simulink model "WindTurbine_TypeIV_HM"  (R2022a)
settings: Solver=FixedStepDiscrete  StartTime=0  StopTime=3  FixedStep=Ts  RelTol=1e-3  EnableMultiTasking=on
InitFcn:
  | load('xInitial_WPP.mat');
  | Ts = 50e-6;
undefined symbols (not defined in the file): D1, Delta, DiscIntNeverNeededParam, LowerLimit, magnitude, UpperLimit
libraries: powerlib x47, simulink x28, powerlib_meascontrol x17, powerlib_extras x6
(part 1 of 2)
settings Model: SimulationMode=accelerator  Creator=ch0272
settings SolverCC: AlgebraicLoopSolver=TrustRegion
settings DataIOCC: FinalStateName=xInitial_WPP  InitialState=xInitial_WPP  LimitDataPoints=on  LoadInitialState=on  SaveFormat=StructureWithTime  SignalLoggingSaveFormat=ModelDataLogs  ReturnWorkspaceOutputs=off
settings OptimizationCC: ExpressionDepthLimit=2147483647  InitFltsAndDblsToZero=on  LifeSpan=inf
settings DebuggingCC: SaveWithParameterizedLinksMsg=none  UnderspecifiedInitializationDetection=Classic  MergeDetectMultiDrivingBlocksExec=none  SignalResolutionControl=TryResolveAllWithWarning  SolverPrmCheckMsg=warning  MultiTaskCondExecSysMsg=none  FcnCallInpInsideContextMsg=warning  StateNameClashWarn=warning  SFUnexpectedBacktrackingDiag=warning  SFNoUnconditionalDefaultTransitionDiag=warning  ArithmeticOperatorsInVariantConditions=warning
settings HardwareCC: ProdBitPerPointer=32  ProdBitPerSizeT=32  ProdBitPerPtrDiffT=32  ProdLargestAtomicFloat=None  ProdIntDivRoundTo=Undefined  ProdEndianess=Unspecified  ProdWordSize=32  ProdHWDeviceType=32-bit Generic  TargetHWDeviceType=32-bit Generic
settings ModelReferenceCC: PropagateSignalLabelsOutOfModel=off
settings SFSimCC: SimUseLocalCustomCode=off  CustomCodeUndefinedFunction=UseInterfaceOnly
settings RTWCC: Description=General HyperLink Target  SystemTargetFile=hyperlink.tlc  TemplateMakefile=hyperlink.tmf  RTWUseLocalCustomCode=off
settings CodeAppCC: StateflowObjectComments=on
settings STFCustomTargetCC: TargetFcnLib=ansi_tfl_tmw.mat  ModelReferenceCompliant=off  CPPClassGenCompliant=on  SystemTargetFile=hyperlink.tlc
settings GRTTargetCC: TargetFcnLib=ansi_tfl_tmw.mat  TargetLangStandard=C89/C90 (ANSI)  ModelReferenceCompliant=off  ParMdlRefBuildCompliant=off  CompOptLevelCompliant=off  ConcurrentExecutionCompliant=off  CombineOutputUpdateFcns=off  MatFileLogging=off  GRTInterface=on  UseToolchainInfoCompliant=off  ExtModeMexFile=noextcomm
settings ConfigComp: CovMetricSettings=dw  CovSaveCumulativeToWorkspaceVar=on  CovSaveSingleToWorkspaceVar=on  CovExternalEMLEnable=off  CovBoundaryAbsTol=1.0e-5
settings SimscapeCC: SimscapeNormalizeSystem=off

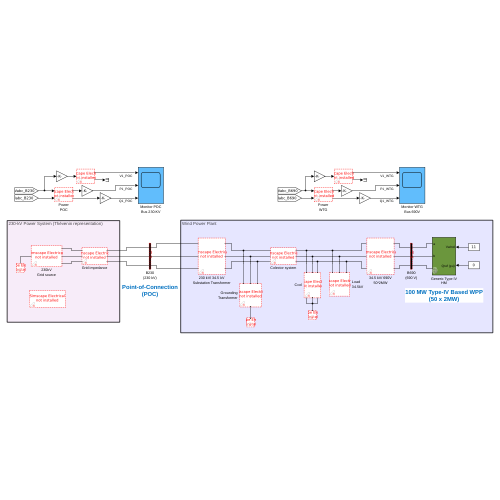
[thumbnail: Simulink's stored preview of the top-level diagram]
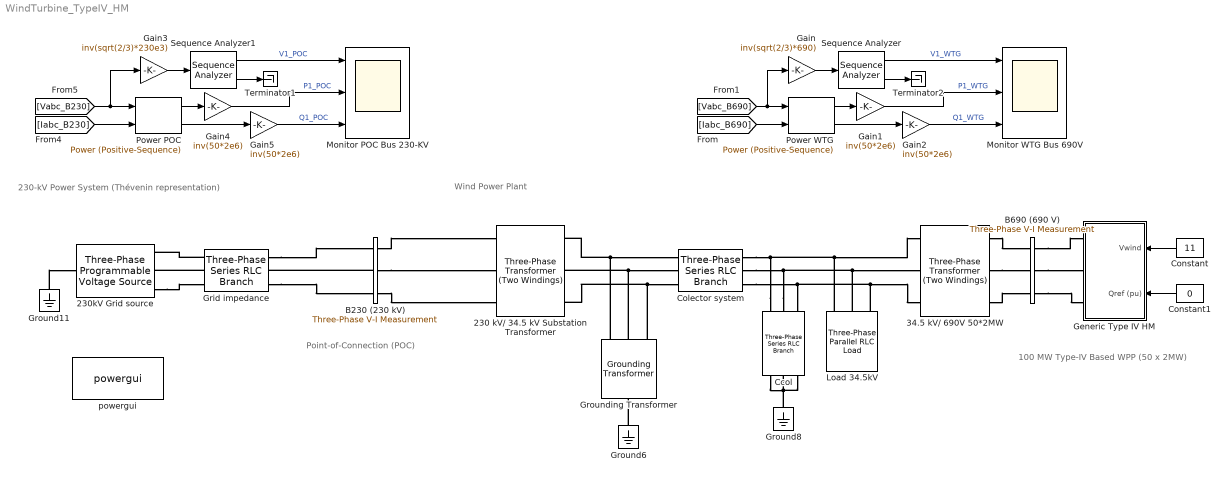
== system WindTurbine_TypeIV_HM ==
  note: 230-kV Power System (Thévenin representation)
  note: Wind Power Plant
  note: 100 MW Type-IV Based WPP
      | (50 x 2MW)
  note: Point-of-Connection
      | (POC)
  230 kV/ 34.5 kV Substation Transformer : powerlib/Elements/Three-Phase Transformer (Two Windings)  Winding1Connection=Yg  Winding2Connection=Delta (D1)  CoreType=Three single-phase transformers  SetSaturation=off  Hysteresis=off  DataFile='hysteresis'  SetInitialFlux=off  Measurements=None  UNITS=pu  NominalPower=[ 115e6 60 ]  Winding1=[230e3 2.25e-3 103.5e-3]  Winding2=[ 34.5e3 0.25e-3 11.5e-3]  Rm=200  Lm=500  L0=0.5  Saturation=[ 0,0 ; 0.002,1 ; 0.01,1.075; 0.025,1.15; 0.05,1.2; 0.1,1.23; 2,1.72 ]  InitialFluxes=[-0.00823815438284101 -0.908209070473327 0.916447224856743]  MoreParameters=off  BreakLoop=off  DataType=off  TransfoNumber=1
  230kV Grid source : powerlib/Electrical Sources/Three-Phase Programmable Voltage Source  PositiveSequence=[230e3 90 60]  VariationEntity=Amplitude  VariationType=Table of time-amplitude pairs  VariationTypeAlt=Step  VariationStep=0.5  VariationRate=10  VariationMagnitude=0.3  VariationFrequency=2  VariationTiming=[1 2]  VariationPhaseA=off  Amplitudes=[1 0.5 1]  TimeValues=[0 1.0 1.1]  HarmonicGeneration=off  HarmonicA=[3 0.2 -25 0]  HarmonicB=[2 0.15 35 2]  Timing="[0.05  3]"  BusType=swing  Pref=0  Qref=0  Qmin=-inf  Qmax=inf
  34.5 kV/ 690V 50*2MW : powerlib/Elements/Three-Phase Transformer (Two Windings)  Winding1Connection=Delta (D1)  Winding2Connection=Yg  CoreType=Three single-phase transformers  SetSaturation=off  Hysteresis=off  DataFile='hysteresis'  SetInitialFlux=off  Measurements=Winding currents  UNITS=pu  NominalPower=[ 115e6 , 60 ]  Winding1=[ 34.5e3 , 3.375e-3 , 51.3e-3]  Winding2=[ 690 , 0.375e-3, 5.7e-3]  Rm=200  Lm=500  L0=0.5  Saturation=[ 0,0 ; 0.002,1 ; 0.01,1.075; 0.025,1.15; 0.05,1.2; 0.1,1.23; 2,1.72 ]  InitialFluxes=[-0.0108935053581042 -0.89679491323339 0.907688418591632]  MoreParameters=off  BreakLoop=off  DataType=off  TransfoNumber=1
  B230 (230 kV) : powerlib/Measurements/Three-Phase V-I Measurement  VoltageMeasurement=phase-to-ground  SetLabelV=on  LabelV=Vabc_B230  Vpu=off  VpuLL=off  CurrentMeasurement=yes  SetLabelI=on  LabelI=Iabc_B230  Ipu=off  Pbase=100e6  Vbase=230e3  OutputType=Complex  PhasorSimulation=off  PSBequivalent=0
  B690 (690 V) : powerlib/Measurements/Three-Phase V-I Measurement  VoltageMeasurement=phase-to-ground  SetLabelV=on  LabelV=Vabc_B690  Vpu=off  VpuLL=off  CurrentMeasurement=yes  SetLabelI=on  LabelI=Iabc_B690  Ipu=off  Pbase=100e6  Vbase=690  OutputType=Complex  PhasorSimulation=off  PSBequivalent=0
  Ccol : powerlib/Elements/Three-Phase Series RLC Branch  LConnTagsString=A|B|C  RConnTagsString=A|B|C  BranchType=C  Resistance=1  Inductance=1e-3  Capacitance=7.17e-6  Measurements=Branch voltages
  Colector system : powerlib/Elements/Three-Phase Series RLC Branch  LConnTagsString=A|B|C  RConnTagsString=A|B|C  BranchType=RL  Resistance=0.22  Inductance=0.391e-3  Capacitance=1e-6  Measurements=Branch currents
  Constant : Constant  Value=11
  Constant1 : Constant  Value=0
  Gain : Gain  Gain=inv(sqrt(2/3)*690)
  Gain{1..2,4..5} (4 alike) : Gain  Gain=inv(50*2e6)
  Gain3 : Gain  Gain=inv(sqrt(2/3)*230e3)
  Generic Type IV HM : Subsystem  mask(WEC Type IV Hybrid Model (HM)){U_rated=690, f_rated=60, FRT_Mode=FRT Mode 1 (I_reactive support), FRT1_triggers=[0.8 1.2 0.01 5], FRT1_k_vrt=[2 2], FRT2_triggers=[0.8 1.2 0.01 5], FRT2_ramp=[0.5 0.2 0], u_protect=[1.25 0.1 0.8 5], f_protect=[1.05 1 0.95 1], Nb_WT=50}
      mask prompts: U_rated "Grid nominal voltage (V):"; f_rated "Grid nominal frequency (Hz):"; FRT_Mode "Fault-ride-through (FRT) Strategy:"; FRT1_triggers "UVRT-trigger, OVRT-trigger, FRT-band (pu) and FRT-maxTime (s):"; FRT1_k_vrt "Proportional gains [k_UVRT k_OVRT]:"; FRT2_triggers "UVRT-trigger, OVRT-trigger, FRT-band (pu) and FRT-maxTime (s):"; FRT2_ramp "P and Q ramp-up times in (s) and start-delay (s):"; u_protect "Voltage protection [Vmax(pu) Vmax_delay(s) Vmin(pu) Vmin_delay(s)]:"; f_protect "Frequency protection [fmax(pu) fmax_delax(s) fmin(pu) fmin_delay(s)]:"; Nb_WT "Number of wind turbines:"
      mask init:
      | %% FRT:
      | if FRT_Mode == 1
      |     u_uvrt = FRT1_triggers(1);
      |     u_ovrt = FRT1_triggers(2);
      |     frt_band = FRT1_triggers(3);
      |     FRT_maxTime = FRT1_triggers(4);
      |     k_uvrt = max(FRT1_k_vrt(1),0); % limit low to 0
      |     k_uvrt = min(FRT1_k_vrt(1),10); % limit max to 10
      |     k_ovrt = max(FRT1_k_vrt(2),0); % limit low to 0
      |     k_ovrt = min(FRT1_k_vrt(2),10); % limit low to 10
      |     FRT2_ramp_p = 0;
      |     FRT2_ramp_q = 0;
      |     FRT2_delay  = 0;
      | elseif FRT_Mode == 2
      |     u_uvrt = FRT2_triggers(1);
      |     u_ovrt = FRT2_triggers(2);
      |     frt_band = FRT2_triggers(3);
      |     FRT_maxTime = FRT2_triggers(4);
      |     FRT2_ramp_p = FRT2_ramp(1);
      |     FRT2_ramp_q = FRT2_ramp(2);
      |     FRT2_delay  = min(FRT2_ramp(3),1); % limt low to 1s
      |     k_uvrt = 0;
      |     k_ovrt = 0;
      | end
      | 
      | %% Protection settings:
      | umax_protection = u_protect(1);
      | umax_delay = u_protect(2);
      | umin_protection = u_protect(3);
      | umin_delay = u_protect(4);
      | fmax_protection = f_protect(1);
      | fmax_delay = f_protect(2);
      | fmin_protection = f_protect(3);
      | fmin_delay = f_protect(4);
      | 
      | %% WEC Parameters:
      | P_rated = 2e6;
      | Q_rated = 1.5e6;
      | i_rated = sqrt(2)*abs((P_rated-j*(Q_rated))/(sqrt(3)*U_rated));
      | i_max = 1.075*i_rated;
      | f_boost = 2e3;
      | f_chopper = 2e3;
      | Vdc_ref = 1250;
      | 
      | %% Generator:
      | % Nominal power, voltage, frequency, field current  [ Pn(VA) Vn(Vrms) fn(Hz) ifn(A) ]:
      | Pgen_nom = 2e6; % [W] 
      | Vgen_nom = 0.83e3; % [V]
      | fgen_nom = 10.8; % [Hz]
      | ifngen_nom = 31.7; % [A]
      | % Stator  [ Rs(ohm)  Ll,Lmd,Lmq(H) ]:
      | Rs_gen = 25e-3; % [Ohm]
      | Ll_gen = 7e-3; % [H]
      | Lmd_gen = 10e-3; % [H]
      | Lmq_gen = 10e-3; % [H]
      | % Field  [ Rf'(ohm)  Llfd'(H) ]:
      | Rf_prime = 3.5e-3; % [Ohm]
      | Llfd_prime = 85e-6; % [H]
      | % Dampers   [ Rkd',Llkd'  Rkq1',Llkq1'  ] (R=ohm,L=H):
      | Rkd_prime = 1e6; % [Ohm]
      | Llkd_prime = 1e-6; % [H]
      | Rkq_prime = 1e6; % [Ohm]
      | Llkq_prime = 1e-6; % [H]
      | % Inertia, friction factor, pole pairs [ J(kg.m^2)  F(N.m.s)  p() ]:
      | J_gen = 7.5e6; % [kgm^2]
      | F_gen = 0; % [Nms]
      | p_gen = 36; % [pole pairs]
      | % Initial conditions  [ dw(%)  th(deg)  ia,ib,ic(A)  pha,phb,phc(deg)  Vf(V) ]:
      | dw_gen = 0; % [%]
      | th_gen = -17.7582; % [deg]
      | ia_gen = 1967.46; % [A]
      | ib_gen = 1967.46; % [A]
      | ic_gen = 1967.46; % [A]
      | pha_gen = 0; % [deg]
      | phb_gen = -120; % [deg]
      | phc_gen = 120; % [deg]
      | Vf_gen = 580; % [V]
      | if0 = 110; % [A]
      | % Load-flow-TAB:
      | Qmax_gen = inf;
      | 
      | %% Universal Bridge (rectifier):
      | Rs_rec = 1e5; % [Ohm]
      | Cs_rec = 1e9; % [F]
      | Ron_rec = 1e-4; % [Ohm]
      | Lon_rec = 0; % [H]
      | Vf_rec = 0; % [V]
      | 
      | %% DC-Link:
      | R1_dc = 1e3; % [Ohm]
      | C1_dc = 50e-3; % [F]
      | C1_V0 = 3*sqrt(2)/pi*830; % [V]
      | R_boost = 10e-3; % [Ohm] 
      | L_boost = 100e-6; % [H]
      | i0_boost = 0; % [A]
      | Ron_igbt_boost = 1e-4; % [Ohm]
      | Lon_igbt_boost = 0; % [H]
      | Vf_igbt_boost = 0; % [V]
      | Rs_igbt_boost = 1e5; % [Ohm]
      | i0_igbt_boost = 0; % [A]
      | Cs_igbt_boost = 1e9; % [F]
      | Ron_diode_boost = 1e-4; % [Ohm]
      | Lon_diode_boost = 0; % [H]
      | Vf_diode_boost = 0; % [V]
      | Rs_diode_boost = 1e5; % [Ohm]
      | Cs_diode_boost = 1e9; % [F]
      | Ron_igbt_chop = 1e-4; % [Ohm]
      | Lon_igbt_chop = 0; % [H]
      | Vf_igbt_chop = 0; % [V]
      | Rs_igbt_chop = 1e5; % [Ohm]
      | Cs_igbt_chop = 1e9; % [F]
      | R_chopper = 0.15; % [Ohm]
      | R2_dc = 1e3; % [Ohm]
      | C2_dc = 0.3; % [F]
      | C2_V0 = 0.9*(Vdc_ref); % [V]
      | Chop_band = 0.025; % [%]
      | 
      | %% Grid Side Converter:
      | Rs_inv = 1e5; % [Ohm]
      | Cs_inv = 1e9; % [F]
      | Ron_inv = 1e-4; % [Ohm]
      | Vf_inv = 0; % [V]
      | Vfd_inv = 0; % [V]
      | 
      | %% Output Filter:
      | L1_filter = 150e-6; % [H]
      | Rshunt_filter = 0.25; % [Ohm]
      | Lshunt_filter = 15e-3; % [H]
      | Cshunt_filter = 1300e-6; % [F]
      | L2_filter = 5e-6; % [H]
      | 
      | %% Three-phase breaker;
      | Ron_breaker = 1e-9; % [Ohm]
      | Rs_breaker = 1e6; % [Ohm]
      | Cs_breaker = 1e9; % [F]
      | 
      | %% Turbine Control:
      | % Rate Limiter (wind speed):
      | v_rise_rate = 5; % m/s
      | v_fall_rate = -5; % m/s
      | v_init = 11;
      | % Pitch_angle:
      | Beta0 = 0; % [deg]
      | % Vdc control:
      | Vdc1_lowLim = 0; % [V]
      | Vdc1_Kp = 0.75; 
      | Vdc1_Ki = 0.075;
      | Vdc1_stateInit = 0.4; 
      | % Wind turbine:
      | R_turb = 42; % [m]
      | ro_air = 1.225; % air density
      | vspeed_max = 11; % [m/s]
      | vspeed_min = 4; % [m/s]
      | lambda_opt = 7.1;
      | w_init = 1.878; % [rad/s]
      | wr_ref_tau = 8; % [s]
      | 
      | %% Extract References:
      | % Measurement Filter (Voltage):
      | f_cut_volt = 10e3; % [Hz]
      | zeta_filt_volt = 1/sqrt(2); % [-]
      | % Measurement Filter (Voltage):
      | f_cut_curr = 10e3; % [Hz]
      | zeta_filt_curr = 1/sqrt(2); % [-]
      | % PLL:
      | pll_Ki = 2.13; % [-]
      | pll_Kp = 0.1775; % [-]
      | 
      | %% Grid-Side Inverter Control:
      | % Vdc2 control:
      | Vdc2_tau = 2*inv(f_rated); % [s]
      | Vdc2_filt_init = C2_V0; % [V]
      | Vdc2_Kp = 10; 
      | Vdc2_Ki = 75; 
      | Vdc2_stateInit = 2000; % [V]
      | % Reactive power control:
      | Q_Kp = 1e-3; % proportional gain
      | Q_Ki = 0.035; % integral gain
      | Q_stateInit = 0; % [V]
      mask Help:
      | Please, refer to work published in:
      | A. S. Trevisan, A. A. El-Deib, R. Gagnon, J. Mahseredjian, and M. Fecteau, “Field Validated Generic EMT-Type Model of a Full Converter Wind Turbine Based on a Gearless Externally Excited Synchronous Generator,” IEEE Trans. Power Deliv., vol. 33, no. 5, pp. 2284–2293, Oct. 2018.
      | 
      | Author: Aramis Schwanka Trevisan
      | aramis.schwanka.trevisan@enercon.de
      mask TypeOptions FRT_Mode: FRT Mode 1 (I_reactive support) | FRT Mode 2 (Zero power mode)
      mask Callback FRT_Mode:
      | BlockName=getfullname(gcb);
      | 
      | Param_Show=get_param(BlockName,'FRT_Mode');
      | Param_Visible=get_param(BlockName,'MaskVisibilities');
      | Param_Visible{3}='on';
      | Param_Visible{4}='off';Param_Visible{5}='off';Param_Visible{6}='off';Param_Visible{7}='off';
      | 
      | switch Param_Show
      | 	case 'FRT Mode 1 (I_reactive support)'
      | 		Param_Visible{4}='on';Param_Visible{5}='on';
      |     case 'FRT Mode 2 (Zero power mode)'
      | 		Param_Visible{6}='on';Param_Visible{7}='on';
      | end
      | 
      | set_param(BlockName,'MaskVisibilities',Param_Visible);
  Grid impedance : powerlib/Elements/Three-Phase Series RLC Branch  LConnTagsString=A|B|C  RConnTagsString=A|B|C  BranchType=RL  Resistance=(230e3^2/800e6)/12.5  Inductance=(230e3^2/800e6)/2/pi/60  Capacitance=1e-6  Measurements=Branch currents
  Ground11 : powerlib/Elements/Ground  LConnTagsString=a
  Ground6 : powerlib/Elements/Ground  LConnTagsString=a
  Ground8 : powerlib/Elements/Ground  LConnTagsString=a
  Grounding Transformer : powerlib/Elements/Grounding Transformer   UNITS=pu  NominalPower="[100e6   60]"  NominalVoltage=34.5e3  ZeroSequenceImpedance_pu=[23.5245 , 630.1197]*1e-3  MagnetizationBranch_pu=[1e6 inf]  ZeroSequenceImpedance_SI=[0.28 7.5]  MagnetizationBranch_SI=[59513 59513]  Measurements=None
  Load 34.5kV : powerlib/Elements/Three-Phase Parallel RLC Load  LConnTagsString=A|B|C  Configuration=Y (grounded)  NominalVoltage=34.5e3  Vabc=[1e3 1e3 1e3]  Vabcp=[1e3 1e3 1e3]  NominalFrequency=60  UnbalancedPower=off  ActivePower=60e3  InductivePower=0  CapacitivePower=0  Pabc=[10e3 9e3 11e3]  QLabc=[100 90 110]  QCabc=[100 90 110]  Pabcp=[10e3 9e3 11e3]  QLabcp=[100 90 110]  QCabcp=[100 90 110]  Measurements=Branch currents  LoadType=constant Z
  Monitor POC Bus 230-KV : Scope  NumInputPorts=3
  Monitor WTG Bus 690V : Scope  NumInputPorts=3
  Power POC : powerlib_meascontrol/Measurements/Power (Positive-Sequence)  Freq=60  Vinit=[0, 0]  Iinit=[0, 0]  Ts=Ts
  Power WTG : powerlib_meascontrol/Measurements/Power (Positive-Sequence)  Freq=60  Vinit=[0, 0]  Iinit=[0, 0]  Ts=Ts
  Sequence Analyzer : powerlib_meascontrol/Measurements/Sequence Analyzer  Freq=60  n=1  seq=Positive  InInit=[1, 0]  Ts=Ts
  Sequence Analyzer1 : powerlib_meascontrol/Measurements/Sequence Analyzer  Freq=60  n=1  seq=Positive  InInit=[1, 0]  Ts=Ts
  Terminator1 : Terminator
  Terminator2 : Terminator
  powergui : powerlib/powergui  SimulationMode=Discrete  SolverType=Tustin  SampleTime=Ts  frequency=60  SPID=off  DisableSnubberDevices=off  DisableRonSwitches=off  DisableVfSwitches=off  SwTol=0  DisplayEquations=off  Interpol=off  ExternalGateDelay=off  methode=off  Ts=0  FunctionMessages=off  echomessages=off  HookPort=off  EnableUseOfTLC=off  x0status=blocks  frequencyindice=0  Pbase=100e6  ErrMax=1e-4  Iterations=50  UnitsV=kV  UnitsW=MW  buscounter=0  RestoreLinks=warning  ResistiveCurrentMeasurement=off  Frange=[1:1:300]  Ylog=off  Xlog=off  ShowGrid=off  save=on  variable=ZData  structure=Vabc_Iabc  ZoomFFT=on  StartTime=0.0  cycles=1  DisplayStyle=1  fundamental=60  FreqAxis=off  MaxFrequency=1000  frequencyindicesteady=1  RmsSteady=1  display=off
  wires:
  Constant1/1 -> Generic Type IV HM/2(Qref (pu))
  Constant/1 -> Generic Type IV HM/1(Vwind)
  [Iabc_B690] -> Power WTG/2
  Power WTG/1 -> Gain1/1
  Power WTG/2 -> Gain2/1
  Sequence Analyzer/2 -> Terminator2/1
  Sequence Analyzer/1 -> Monitor WTG Bus 690V/1  "V1_WTG"
  [Vabc_B690] -> Gain/1, Power WTG/1
  Power POC/1 -> Gain4/1
  Power POC/2 -> Gain5/1
  Sequence Analyzer1/2 -> Terminator1/1
  Sequence Analyzer1/1 -> Monitor POC Bus 230-KV/1  "V1_POC"
  [Vabc_B230] -> Gain3/1, Power POC/1
  [Iabc_B230] -> Power POC/2
  Gain/1 -> Sequence Analyzer/1
  Gain1/1 -> Monitor WTG Bus 690V/2  "P1_WTG"
  Gain2/1 -> Monitor WTG Bus 690V/3  "Q1_WTG"
  Gain3/1 -> Sequence Analyzer1/1
  Gain4/1 -> Monitor POC Bus 230-KV/2  "P1_POC"
  Gain5/1 -> Monitor POC Bus 230-KV/3  "Q1_POC"
  connections:
  Grounding Transformer/LConn1 -- Colector system/RConn1 -- 230 kV/ 34.5 kV Substation Transformer/RConn1
  Ccol/RConn3 -- Ccol/RConn2 -- Ground8/LConn1 -- Ccol/RConn1
  Grounding Transformer/LConn2 -- Colector system/RConn2 -- 230 kV/ 34.5 kV Substation Transformer/RConn2
  Grounding Transformer/LConn3 -- Colector system/RConn3 -- 230 kV/ 34.5 kV Substation Transformer/RConn3
  Load 34.5kV/LConn3 -- Colector system/LConn3 -- Ccol/LConn3 -- 34.5 kV/ 690V 50*2MW/LConn3
  Ccol/LConn2 -- Load 34.5kV/LConn2 -- 34.5 kV/ 690V 50*2MW/LConn2 -- Colector system/LConn2
  Ccol/LConn1 -- Load 34.5kV/LConn1 -- 34.5 kV/ 690V 50*2MW/LConn1 -- Colector system/LConn1
  Ground11/LConn1 -- 230kV Grid source/LConn1
  B690 (690 V)/LConn2 -- Generic Type IV HM/RConn2
  B690 (690 V)/LConn1 -- Generic Type IV HM/RConn1
  B690 (690 V)/LConn3 -- Generic Type IV HM/RConn3
  Ground6/LConn1 -- Grounding Transformer/RConn1
  B230 (230 kV)/LConn2 -- 230 kV/ 34.5 kV Substation Transformer/LConn2
  B230 (230 kV)/LConn1 -- 230 kV/ 34.5 kV Substation Transformer/LConn1
  B230 (230 kV)/LConn3 -- 230 kV/ 34.5 kV Substation Transformer/LConn3
  34.5 kV/ 690V 50*2MW/RConn2 -- B690 (690 V)/RConn2
  34.5 kV/ 690V 50*2MW/RConn1 -- B690 (690 V)/RConn1
  34.5 kV/ 690V 50*2MW/RConn3 -- B690 (690 V)/RConn3
  Grid impedance/RConn2 -- 230kV Grid source/RConn2
  Grid impedance/RConn1 -- 230kV Grid source/RConn1
  230kV Grid source/RConn3 -- Grid impedance/RConn3
  Grid impedance/LConn1 -- B230 (230 kV)/RConn1
  B230 (230 kV)/RConn2 -- Grid impedance/LConn2
  Grid impedance/LConn3 -- B230 (230 kV)/RConn3

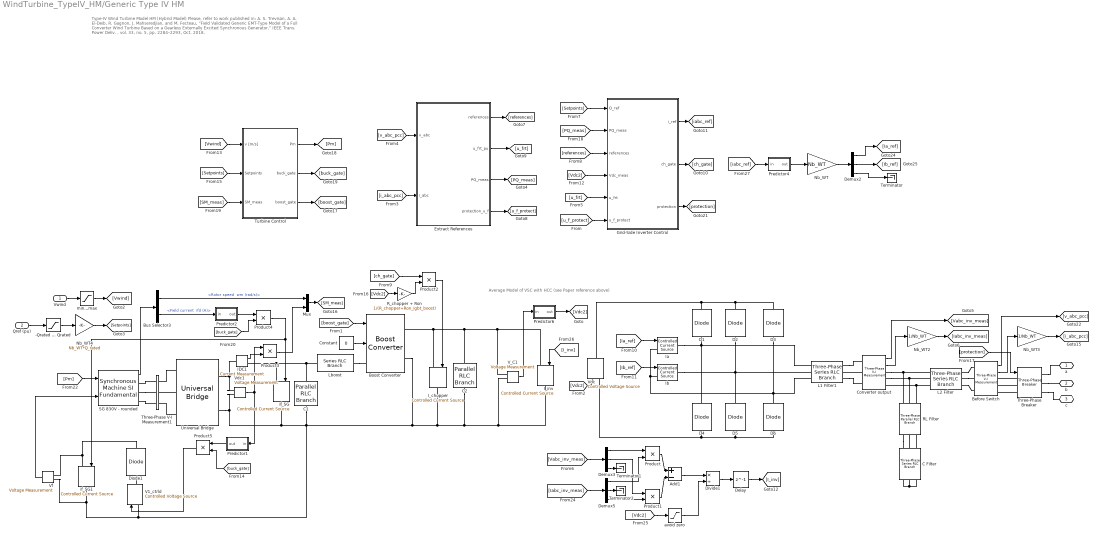
== system WindTurbine_TypeIV_HM/Generic Type IV HM ==
  note: Average Model of VSC with HCC (see Paper reference above)
  note: Type-IV Wind Turbine Model
      | HM (Hybrid Model)
      |
      | Please, refer to work published in:
      |
      | A. S. Trevisan, A. A. El-Deib, R. Gagnon, J. Mahseredjian, and M. Fecteau, “Field Validated Generic EMT-Type Model of a Full Converter Wind Turbine Based on a Gearless Externally Excited Synchronous Generator,” IEEE Trans. Power Deliv. , vol. 33, no. 5, pp. 2284–2293, Oct. 2018.
  Vwind : Inport
  Qref (pu) : Inport  Port=2
  -Qrated ... Qrated : Saturate  UpperLimit=1  LowerLimit=-1
  Add1 : Sum  Inputs=+-
  Before Switch : powerlib/Measurements/Three-Phase V-I Measurement  VoltageMeasurement=phase-to-ground  SetLabelV=off  LabelV=Vabc  Vpu=off  VpuLL=off  CurrentMeasurement=yes  SetLabelI=off  LabelI=Iabc  Ipu=off  Pbase=100e6  Vbase=500e3  OutputType=Complex  PhasorSimulation=off  PSBequivalent=0
  Boost Converter : powerlib/Power Electronics/Boost Converter  ModelType=Switching function  Ron=1e-3  Rs=1e6  Cs=inf  Vforward=[0,0]  Ron_Diode=Ron_diode_boost  Rs_Diode=Rs_diode_boost  Cs_Diode=Cs_diode_boost  Vf_Diode=Vf_diode_boost  Rs_CurrentSource=1e5
  Bus Selector3 : BusSelector  OutputSignals="Mechanical.Rotor speed  wm (rad/s),dq0 components.Field current  ifd (A)"
  C Filter : powerlib/Elements/Three-Phase Series RLC Branch  LConnTagsString=A|B|C  RConnTagsString=A|B|C  BranchType=C  Resistance=1  Inductance=50e-6  Capacitance=Cshunt_filter*Nb_WT  Measurements=Branch voltages
  C1 : powerlib/Elements/Parallel RLC Branch  LConnTagsString=a  RConnTagsString=__new0  BranchType=C  Resistance=R1_dc  Inductance=1e-3  SetiL0=off  InitialCurrent=0  Capacitance=C1_dc  Setx0=on  InitialVoltage=C1_V0  Measurements=None
  C2 : powerlib/Elements/Parallel RLC Branch  LConnTagsString=a  RConnTagsString=__new0  BranchType=C  Resistance=R2_dc  Inductance=1e-3  SetiL0=off  InitialCurrent=0  Capacitance=C2_dc  Setx0=on  InitialVoltage=C2_V0  Measurements=None
  Constant : Constant  Value=0
  Converter output : powerlib/Measurements/Three-Phase V-I Measurement  VoltageMeasurement=phase-to-phase  SetLabelV=off  LabelV=Vabc  Vpu=off  VpuLL=off  CurrentMeasurement=yes  SetLabelI=off  LabelI=Iabc  Ipu=off  Pbase=100e6  Vbase=500e3  OutputType=Complex  PhasorSimulation=off  PSBequivalent=0
  D{1..6} (6 alike) : powerlib/Power Electronics/Diode  Ron=Ron_inv/Nb_WT  Lon=0  Vf=Vfd_inv  IC=0  UseSnubber=off  Rs=Rs_inv/Nb_WT  Cs=Cs_inv*Nb_WT  Measurements=off
  Delay : Delay  DelayLength=1  SampleTime=Ts
  Demux2 : Demux  Outputs=3
  Demux3 : Demux  Outputs=3
  Demux5 : Demux  Outputs=3
  Diode1 : powerlib/Power Electronics/Diode  Ron=1e-3  Lon=0  Vf=0  IC=0  UseSnubber=off  Rs=1e5  Cs=250e-9  Measurements=off
  Divide1 : Product  Inputs=*/
  Extract References : Subsystem
  Grid-Side Inverter Control : Subsystem
  IDC1 : powerlib/Measurements/Current Measurement  PhasorSimulation=off  OutputType=Complex  PSBequivalent=0
  I_chopper : powerlib/Electrical Sources/Controlled Current Source  Initialize=on  Source_Type=AC  Amplitude=0  Phase=0  Frequency=0  Measurements=None
  I_inv : powerlib/Electrical Sources/Controlled Current Source  Initialize=on  Source_Type=AC  Amplitude=0  Phase=0  Frequency=0  Measurements=None
  Ia : powerlib/Electrical Sources/Controlled Current Source  Initialize=on  Source_Type=AC  Amplitude=0  Phase=0  Frequency=0  Measurements=None
  Ib : powerlib/Electrical Sources/Controlled Current Source  Initialize=on  Source_Type=AC  Amplitude=0  Phase=0  Frequency=0  Measurements=None
  L1 Filter1 : powerlib/Elements/Three-Phase Series RLC Branch  LConnTagsString=A|B|C  RConnTagsString=A|B|C  BranchType=L  Resistance=1  Inductance=L1_filter/Nb_WT  Capacitance=1e-6  Measurements=None
  L2 Filter : powerlib/Elements/Three-Phase Series RLC Branch  LConnTagsString=A|B|C  RConnTagsString=A|B|C  BranchType=L  Resistance=1  Inductance=L2_filter/Nb_WT  Capacitance=1e-6  Measurements=None
  Lboost : powerlib/Elements/Series RLC Branch  LConnTagsString=__new0  RConnTagsString=__new0  BranchType=RL  Resistance=R_boost  Inductance=L_boost  SetiL0=on  InitialCurrent=i0_boost  Capacitance=100e-6  Setx0=on  InitialVoltage=350  Measurements=None
  Mux : Mux  Inputs=2
  Nb_WT : Gain  Gain=Nb_WT
  Nb_WT2 : Gain  Gain=1/Nb_WT
  Nb_WT3 : Gain  Gain=1/Nb_WT
  Nb_WT4 : Gain  Gain=Nb_WT*Q_rated
  Predictor1 : Subsystem  mask{Init_value=3*sqrt(2)/pi*830, Ts=Ts}
      mask prompts: Init_value "Initial value:"; Ts "Sample time (Ts):"
  Predictor2 : Subsystem  mask{Init_value=if0, Ts=Ts}
      mask prompts: Init_value "Initial value:"; Ts "Sample time (Ts):"
  Predictor4 : Subsystem  mask{Init_value=0, Ts=Ts}
      mask prompts: Init_value "Initial value:"; Ts "Sample time (Ts):"
  Predictor6 : Subsystem  mask{Init_value=0.9*(Vdc_ref), Ts=Ts}
      mask prompts: Init_value "Initial value:"; Ts "Sample time (Ts):"
  Product{,1..5} (6 alike) : Product
  RL Filter : powerlib/Elements/Three-Phase Parallel RLC Branch  LConnTagsString=A|B|C  RConnTagsString=A|B|C  BranchType=RL  Resistance=Rshunt_filter/Nb_WT  Inductance=Lshunt_filter/Nb_WT  Capacitance=1e-6  Measurements=Branch currents
  R_chopper + Ron : Gain  Gain=1/(R_chopper+Ron_igbt_boost)
  SG 830V - rounded : powerlib/Machines/Synchronous Machine SI Fundamental  PresetModel=No  MechanicalLoad=Mechanical power Pm  ShowDetailedParameters=on  RotorType=Salient-pole  Units=SI fundamental parameters  MeasurementBus=off  NominalParameters="[ Pgen_nom  Vgen_nom  fgen_nom  ifngen_nom]"  Stator=[ Rs_gen Ll_gen Lmd_gen Lmq_gen ]  Field=[ Rf_prime Llfd_prime ]  Dampers2=[ 0.0664, 1.387e-3, 0.0292, 6.896e-4, 7.907e-3, 2.477e-3]  Dampers1=[ Rkd_prime Llkd_prime Rkq_prime Llkq_prime ]  Mechanical=[ J_gen F_gen p_gen ]  PolePairs=36  InitialConditions=[ dw_gen th_gen ia_gen ib_gen ic_gen pha_gen phb_gen phc_gen Vf_gen ]  SetSaturation=off  Saturation=[695.64,774.7,917.5,1001.6,1082.2,1175.9,1293.6,1430.2,1583.7;9660,10623,12243,13063,13757,14437,15180,15890,16567]  DisplayVfd=off  LoadFlowParameters=[2 2000000 0 0 0]  TsPowergui=0  TsBlock=Ts  IterativeModel=Trapezoidal non iterative  IterativeDiscreteModel=Trapezoidal non iterative  BusType=swing  Pref=0  Qref=0  Qmin=-inf  Qmax=Qmax_gen  PLF=0  QLF=0
  Terminator : Terminator
  Terminator1 : Terminator
  Terminator2 : Terminator
  Three-Phase V-I Measurement1 : powerlib/Measurements/Three-Phase V-I Measurement  VoltageMeasurement=no  SetLabelV=off  LabelV=Vabc  Vpu=off  VpuLL=off  CurrentMeasurement=no  SetLabelI=off  LabelI=Iabc  Ipu=off  Pbase=100e6  Vbase=830  OutputType=Complex  PhasorSimulation=off  PSBequivalent=0
  Three-Phase Breaker : powerlib/Elements/Three-Phase Breaker  InitialState=closed  SwitchA=on  SwitchB=on  SwitchC=on  SwitchTimes=[1000]  External=on  BreakerResistance=Ron_breaker/Nb_WT  SnubberResistance=Rs_breaker/Nb_WT  SnubberCapacitance=Cs_breaker*Nb_WT  Measurements=None
  Turbine Control : Subsystem
  Universal Bridge : powerlib/Power Electronics/Universal Bridge  Arms=3  SnubberResistance=Rs_rec  SnubberCapacitance=Cs_rec  Device=Diodes  Ron=Ron_rec  Lon=Lon_rec  ForwardVoltages="[  0  0  ]"  ForwardVoltage=Vf_rec  GTOparameters=[ 10e-6 , 20e-6 ]  IGBTparameters=[ 1e-6 , 2e-6 ]  Measurements=None  Measurements_2=None  converterType=Rectifier
  V1_ctrld : powerlib/Electrical Sources/Controlled Voltage Source  Initialize=on  Source_Type=AC  Amplitude=0  Phase=0  Frequency=0  Measurements=None
  V_C1 : powerlib/Measurements/Voltage Measurement  PhasorSimulation=off  OutputType=Complex  PSBequivalent=0
  Vdc : powerlib/Electrical Sources/Controlled Voltage Source  Initialize=on  Source_Type=AC  Amplitude=0  Phase=0  Frequency=0  Measurements=None
  Vdc1 : powerlib/Measurements/Voltage Measurement  PhasorSimulation=off  OutputType=Complex  PSBequivalent=0
  Vf : powerlib/Measurements/Voltage Measurement  PhasorSimulation=off  OutputType=Complex  PSBequivalent=0
  avoid zero : Saturate  UpperLimit=inf  LowerLimit=1e-6
  if_SG : powerlib/Electrical Sources/Controlled Current Source  Initialize=on  Source_Type=AC  Amplitude=0  Phase=0  Frequency=0  Measurements=None
  if_SG1 : powerlib/Electrical Sources/Controlled Current Source  Initialize=on  Source_Type=AC  Amplitude=0  Phase=0  Frequency=0  Measurements=None
  min...max : Saturate  UpperLimit=11  LowerLimit=4
  a : PMIOPort  Side=Right
  b : PMIOPort  Port=2  Side=Right
  c : PMIOPort  Port=3  Side=Right
  wires:
  [Pm] -> SG 830V - rounded/1
  Bus Selector3/1 -> Mux/1  "<Rotor speed  wm (rad/s)>"
  SG 830V - rounded/1 -> Bus Selector3/1
  Vwind/1 -> min...max/1
  Before Switch/2 -> Nb_WT3/1
  [Vdc2] -> Vdc/1
  [Ia_ref] -> Ia/1
  [Ib_ref] -> Ib/1
  V_C1/1 -> Predictor6/1(in)
  [I_inv] -> I_inv/1
  Demux2/2 -> [Ib_ref]
  Demux2/1 -> [Ia_ref]
  Demux2/3 -> Terminator/1
  [Vabc_inv_meas] -> Demux3/1
  [Iabc_inv_meas] -> Demux5/1
  Product1/1 -> Add1/2
  Product/1 -> Add1/1
  [Vdc2] -> avoid zero/1
  [boost_gate] -> Boost Converter/1
  Constant/1 -> Boost Converter/2
  avoid zero/1 -> Divide1/2
  Before Switch/1 -> [v_abc_pcc]
  Demux3/3 -> Terminator1/1
  Demux5/2 -> Terminator2/1
  Demux5/3 -> Product1/2
  Demux3/2 -> Product1/1
  Demux3/1 -> Product/1
  Demux5/1 -> Product/2
  [iabc_ref] -> Predictor4/1(in)
  [PQ_meas] -> Grid-Side Inverter Control/2(PQ_meas)
  Grid-Side Inverter Control/2(ch_gate) -> [ch_gate]
  [u_frt] -> Grid-Side Inverter Control/5(u_frt)
  [Vdc2] -> Grid-Side Inverter Control/4(Vdc_meas)
  Grid-Side Inverter Control/1(i_ref) -> [iabc_ref]
  [references] -> Grid-Side Inverter Control/3(references)
  [Setpoints] -> Grid-Side Inverter Control/1(Q_ref)
  [v_abc_pcc] -> Extract References/1(v_abc)
  [i_abc_pcc] -> Extract References/2(i_abc)
  Extract References/2(u_frt_pu) -> [u_frt]
  Extract References/3(PQ_meas) -> [PQ_meas]
  Extract References/1(references) -> [references]
  [SM_meas] -> Turbine Control/3(SM_meas)
  [Vwind] -> Turbine Control/1(v [m/s])
  Turbine Control/1(Pm) -> [Pm]
  Turbine Control/2(buck_gate) -> [buck_gate]
  [Setpoints] -> Turbine Control/2(Setpoints)
  IDC1/1 -> Product3/2
  Mux/1 -> [SM_meas]
  Product3/1 -> Mux/2
  [Vdc2] -> R_chopper + Ron/1
  R_chopper + Ron/1 -> Product2/2
  [ch_gate] -> Product2/1
  Product2/1 -> I_chopper/1
  Turbine Control/3(boost_gate) -> [boost_gate]
  Predictor6/1(out) -> [Vdc2]
  Converter output/2 -> Nb_WT2/1
  Converter output/1 -> [Vabc_inv_meas]
  Extract References/4(protection_u_f) -> [u_f_protect]
  [protection] -> Three-Phase Breaker/1
  [u_f_protect] -> Grid-Side Inverter Control/6(u_f_protect)
  Grid-Side Inverter Control/3(protection) -> [protection]
  Bus Selector3/2 -> Predictor2/1(in)  "<Field current  ifd (A)>"
  Predictor2/1(out) -> Product4/1
  [buck_gate] -> Product4/2
  min...max/1 -> [Vwind]
  Vdc1/1 -> Predictor1/1(in), Product3/1
  [buck_gate] -> Product5/2
  Product5/1 -> V1_ctrld/1
  Vf/1 -> SG 830V - rounded/2
  Product4/1 -> if_SG1/1, if_SG/1
  Predictor1/1(out) -> Product5/1
  Predictor4/1(out) -> Nb_WT/1
  Nb_WT/1 -> Demux2/1
  Nb_WT2/1 -> [Iabc_inv_meas]
  Nb_WT3/1 -> [i_abc_pcc]
  Add1/1 -> Divide1/1
  Divide1/1 -> Delay/1
  Delay/1 -> [I_inv]
  Nb_WT4/1 -> [Setpoints]
  Qref (pu)/1 -> -Qrated ... Qrated/1
  -Qrated ... Qrated/1 -> Nb_WT4/1
  connections:
  Vdc1/LConn1 -- Universal Bridge/RConn1 -- IDC1/LConn1
  SG 830V - rounded/RConn3 -- Three-Phase V-I Measurement1/LConn3
  Universal Bridge/LConn2 -- Three-Phase V-I Measurement1/RConn2
  Universal Bridge/LConn1 -- Three-Phase V-I Measurement1/RConn1
  Universal Bridge/LConn3 -- Three-Phase V-I Measurement1/RConn3
  SG 830V - rounded/RConn1 -- Three-Phase V-I Measurement1/LConn1
  SG 830V - rounded/RConn2 -- Three-Phase V-I Measurement1/LConn2
  IDC1/RConn1 -- if_SG/LConn1 -- Lboost/LConn1 -- C1/LConn1
  V_C1/LConn1 -- I_inv/LConn1 -- C2/LConn1 -- I_chopper/LConn1 -- Boost Converter/RConn1
  D3/RConn1 -- D2/RConn1 -- Vdc/RConn1 -- D1/RConn1
  Vdc/LConn1 -- D4/LConn1 -- D6/LConn1 -- D5/LConn1
  Three-Phase Breaker/LConn3 -- Before Switch/RConn3
  Three-Phase Breaker/RConn3 -- c/RConn1
  D5/RConn1 -- L1 Filter1/LConn2 -- D2/LConn1 -- Ib/RConn1
  L2 Filter/LConn3 -- Converter output/RConn3 -- RL Filter/LConn3
  Converter output/RConn2 -- L2 Filter/LConn2 -- RL Filter/LConn2
  Three-Phase Breaker/LConn1 -- Before Switch/RConn1
  Three-Phase Breaker/LConn2 -- Before Switch/RConn2
  Three-Phase Breaker/RConn1 -- a/RConn1
  Three-Phase Breaker/RConn2 -- b/RConn1
  Converter output/RConn1 -- L2 Filter/LConn1 -- RL Filter/LConn1
  I_inv/RConn1 -- C2/RConn1 -- Vdc1/LConn2 -- Universal Bridge/RConn2 -- if_SG/RConn1 -- if_SG1/RConn1 -- Vf/LConn2 -- V1_ctrld/LConn1 -- C1/RConn1 -- Boost Converter/RConn2 -- I_chopper/RConn1 -- V_C1/LConn2
  Lboost/RConn1 -- Boost Converter/LConn1
  C Filter/RConn1 -- C Filter/RConn2 -- C Filter/RConn3
  RL Filter/RConn1 -- C Filter/LConn1
  Converter output/LConn2 -- L1 Filter1/RConn2
  L1 Filter1/RConn1 -- Converter output/LConn1
  L1 Filter1/RConn3 -- Converter output/LConn3
  V1_ctrld/RConn1 -- Diode1/LConn1
  if_SG1/LConn1 -- Vf/LConn1 -- Diode1/RConn1
  Ia/RConn1 -- L1 Filter1/LConn1 -- D4/RConn1 -- D1/LConn1
  D6/RConn1 -- L1 Filter1/LConn3 -- D3/LConn1 -- Ia/LConn1 -- Ib/LConn1
  L2 Filter/RConn2 -- Before Switch/LConn2
  L2 Filter/RConn1 -- Before Switch/LConn1
  L2 Filter/RConn3 -- Before Switch/LConn3
  C Filter/LConn2 -- RL Filter/RConn2
  C Filter/LConn3 -- RL Filter/RConn3

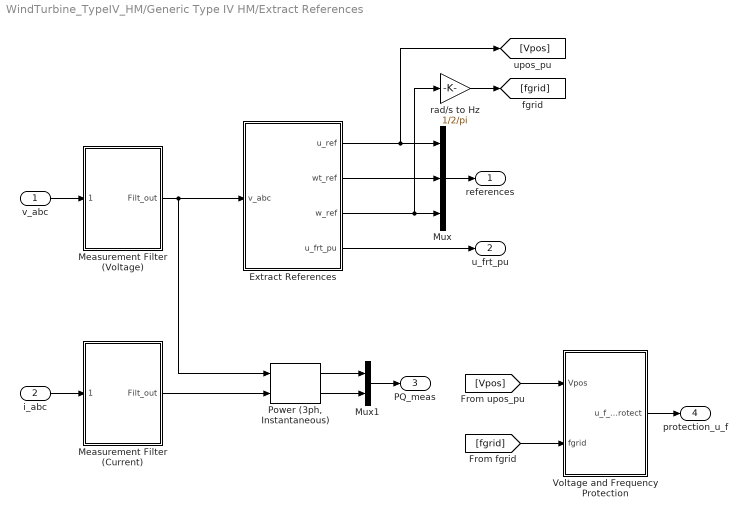
== system WindTurbine_TypeIV_HM/Generic Type IV HM/Extract References ==
  v_abc : Inport
  i_abc : Inport  Port=2
  Extract References : Subsystem
  Measurement Filter (Current) : Subsystem  mask{Freq=f_cut_curr, Zeta=zeta_filt_curr, Ts=Ts}
      mask prompts: Freq "Cut-off frequency (Hz):"; Zeta "Damping factor Zeta (Q=1/(2*Zeta)):"; Ts "Sample time:"
  Measurement Filter (Voltage) : Subsystem  mask{Freq=f_cut_volt, Zeta=zeta_filt_volt, Ts=Ts}
      mask prompts: Freq "Cut-off frequency (Hz):"; Zeta "Damping factor Zeta (Q=1/(2*Zeta)):"; Ts "Sample time:"
  Mux : Mux  Inputs=3
  Mux1 : Mux  Inputs=2
  "Power (3ph, Instantaneous)" : powerlib_meascontrol/Measurements/Power (3ph, Instantaneous)
  Voltage and Frequency Protection : Subsystem
  rad/s to Hz : Gain  Gain=1/2/pi
  references : Outport
  u_frt_pu : Outport  Port=2
  PQ_meas : Outport  Port=3
  protection_u_f : Outport  Port=4
  wires:
  Extract References/4(u_frt_pu) -> u_frt_pu/1
  Extract References/2(wt_ref) -> Mux/2
  Extract References/3(w_ref) -> rad/s to Hz/1, Mux/3
  Mux/1 -> references/1
  "Power (3ph, Instantaneous)"/1 -> Mux1/1
  "Power (3ph, Instantaneous)"/2 -> Mux1/2
  Mux1/1 -> PQ_meas/1
  [Vpos] -> Voltage and Frequency Protection/1(Vpos)
  [fgrid] -> Voltage and Frequency Protection/2(fgrid)
  Voltage and Frequency Protection/1(u_f_protect) -> protection_u_f/1
  Extract References/1(u_ref) -> [Vpos], Mux/1
  rad/s to Hz/1 -> [fgrid]
  v_abc/1 -> Measurement Filter (Voltage)/1(Meas_in)
  Measurement Filter (Voltage)/1(Filt_out) -> Extract References/1(v_abc), "Power (3ph, Instantaneous)"/1
  i_abc/1 -> Measurement Filter (Current)/1(Meas_in)
  Measurement Filter (Current)/1(Filt_out) -> "Power (3ph, Instantaneous)"/2

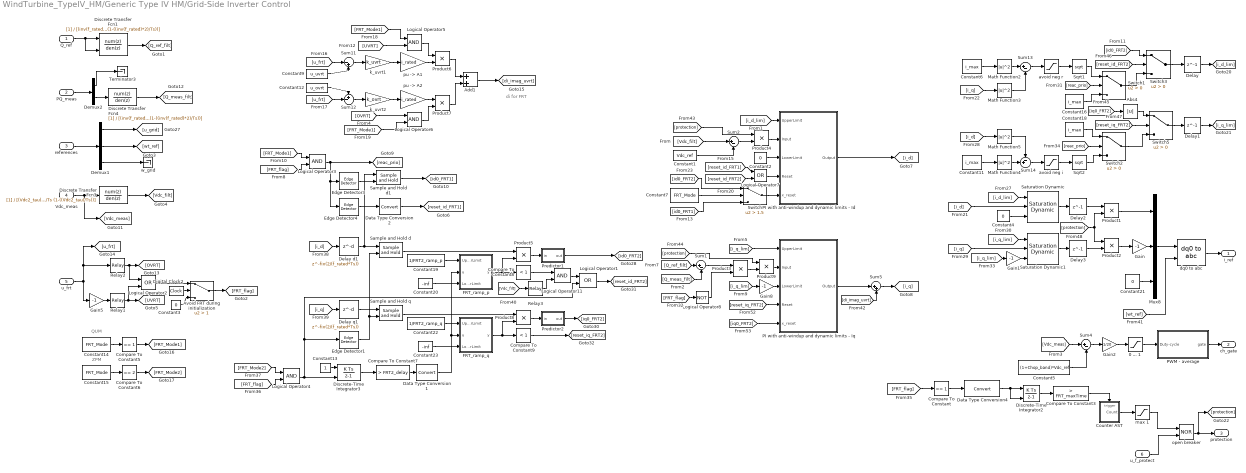
== system WindTurbine_TypeIV_HM/Generic Type IV HM/Grid-Side Inverter Control ==
  note: ZPM
  note: QUM
  note: di for FRT
  Q_ref : Inport
  PQ_meas : Inport  Port=2
  references : Inport  Port=3
  Vdc_meas : Inport  Port=4
  u_frt : Inport  Port=5
  u_f_protect : Inport  Port=6
  0 ... 1 : Saturate  UpperLimit=1  LowerLimit=0
  Abs4 : Abs  SaturateOnIntegerOverflow=off
  Add1 : Sum
  Avoid FRT during initialization : Switch  Criteria=u2 > Threshold  Threshold=1  SaturateOnIntegerOverflow=off  InputSameDT=off
  Compare To Constant : simulink/Logic and Bit Operations/Compare To Constant  relop===  const=1  OutDataTypeStr=boolean
  Compare To Constant3 : simulink/Logic and Bit Operations/Compare To Constant  relop=>  const=FRT_maxTime  OutDataTypeStr=boolean
  Compare To Constant5 : simulink/Logic and Bit Operations/Compare To Constant  relop===  const=1  OutDataTypeStr=boolean
  Compare To Constant6 : simulink/Logic and Bit Operations/Compare To Constant  relop===  const=2  OutDataTypeStr=boolean
  Compare To Constant7 : simulink/Logic and Bit Operations/Compare To Constant  relop=>  const=FRT2_delay  OutDataTypeStr=boolean
  Compare To Constant8 : simulink/Logic and Bit Operations/Compare To Constant  relop=<  const=1  OutDataTypeStr=boolean
  Compare To Constant9 : simulink/Logic and Bit Operations/Compare To Constant  relop=<  const=1  OutDataTypeStr=boolean
  Constant1 : Constant  Value=Vdc_ref  SampleTime=Ts
  Constant{6,11,16,18} (4 alike) : Constant  Value=i_max  SampleTime=Ts
  Constant12 : Constant  Value=u_ovrt  SampleTime=Ts
  Constant13 : Constant
  Constant14 : Constant  Value=FRT_Mode  SampleTime=Ts
  Constant15 : Constant  Value=FRT_Mode  SampleTime=Ts
  Constant19 : Constant  Value=1/FRT2_ramp_p  SampleTime=Ts
  Constant2 : Constant  Value=0  SampleTime=Ts
  Constant20 : Constant  Value=-inf  SampleTime=Ts
  Constant21 : Constant  Value=0  SampleTime=Ts
  Constant22 : Constant  Value=1/FRT2_ramp_q  SampleTime=Ts
  Constant23 : Constant  Value=-inf  SampleTime=Ts
  Constant3 : Constant  Value=0
  Constant4 : Constant  Value=0  SampleTime=Ts
  Constant5 : Constant  Value=(1+Chop_band)*Vdc_ref  SampleTime=Ts
  Constant7 : Constant  Value=FRT_Mode  SampleTime=Ts
  Constant9 : Constant  Value=u_uvrt  SampleTime=Ts
  Counter AST : Subsystem
  Data Type Conversion1 : DataTypeConversion  SaturateOnIntegerOverflow=off  RndMeth=Floor
  Data Type Conversion2 : DataTypeConversion  SaturateOnIntegerOverflow=off  RndMeth=Floor
  Data Type Conversion4 : DataTypeConversion  SaturateOnIntegerOverflow=off  RndMeth=Floor
  Delay{,1..3} (4 alike) : Delay  DelayLength=1  InitialCondition=0  SampleTime=Ts
  Delay d1 : Delay  DelayLength=fix(2/(f_rated*Ts))  InitialCondition=1  SampleTime=Ts
  Delay q1 : Delay  DelayLength=fix(2/(f_rated*Ts))  InitialCondition=1  SampleTime=Ts
  Demux1 : Demux  Outputs=3
  Demux2 : Demux  Outputs=2
  Digital Clock2 : DigitalClock  SampleTime=Ts
  Discrete Transfer Fcn1 : DiscreteTransferFcn  Denominator=[(inv(f_rated)*2)/Ts (1-((inv(f_rated)*2)/Ts))]  InitialStatesSource=Input port  SampleTime=Ts
      settings: InputPortMap=u0,p5
  Discrete Transfer Fcn3 : DiscreteTransferFcn  Denominator=[(Vdc2_tau)/Ts (1-((Vdc2_tau)/Ts))]  InitialStates=Vdc2_filt_init  SampleTime=Ts
  Discrete Transfer Fcn4 : DiscreteTransferFcn  Denominator=[(inv(f_rated)*2)/Ts (1-((inv(f_rated)*2)/Ts))]  InitialStates=U_rated^2/(-inv(2*pi*f_rated*Cshunt_filter))  SampleTime=Ts
  Discrete-Time Integrator2 : DiscreteIntegrator  ExternalReset=falling  SampleTime=Ts  ICPrevOutput=DiscIntNeverNeededParam  ICPrevScaledInput=DiscIntNeverNeededParam
  Discrete-Time Integrator3 : DiscreteIntegrator  ExternalReset=level  SampleTime=Ts  LimitOutput=on  UpperSaturationLimit=1  LowerSaturationLimit=0  ICPrevOutput=DiscIntNeverNeededParam  ICPrevScaledInput=DiscIntNeverNeededParam
  Edge Detector1 : powerlib_meascontrol/Logic/Edge Detector  model=Rising  ic=0  Ts=Ts
  Edge Detector3 : powerlib_meascontrol/Logic/Edge Detector  model=Rising  ic=0  Ts=Ts
  Edge Detector4 : powerlib_meascontrol/Logic/Edge Detector  model=Falling  ic=0  Ts=Ts
  FRT_ramp_p : Subsystem
  FRT_ramp_q : Subsystem
  Gain{,1,5,8} (4 alike) : Gain  Gain=-1
  Gain2 : Gain  Gain=1/20
  Logical Operator1 : Logic  Operator=OR  AllPortsSameDT=off  OutDataTypeStr=boolean
  Logical Operator{3..6,11} (5 alike) : Logic  AllPortsSameDT=off  OutDataTypeStr=boolean
  Logical Operator2 : Logic  Operator=OR  AllPortsSameDT=off  OutDataTypeStr=boolean
  Logical Operator7 : Logic  Operator=OR  AllPortsSameDT=off  OutDataTypeStr=boolean
  Logical Operator8 : Logic  Operator=NOT  AllPortsSameDT=off  OutDataTypeStr=boolean
  Math Function{2..5} (4 alike) : Math  Operator=magnitude^2  SignedPower=on
  Mux8 : Mux  Inputs=3
  PI with anti-windup and dynamic limits - Id : Subsystem  mask(Discrete PI Controller with anti-windup and dynamic limiters){Kp=Vdc2_Kp, Ki=Vdc2_Ki, Init=Vdc2_stateInit, Ts=Ts}
      mask prompts: Kp "Proportional gain (Kp):"; Ki "Integral gain (Ki):"; Init "State initial value:"; Ts "Sample time:"
      mask Display:
      | disp('PI-\nAST');
      | port_label('input',1,'Max');
      | port_label('input',2,'In');
      | port_label('input',3,'Min');
      | port_label('input',4,'Reset');
      | port_label('input',5,'x_reset');
      | port_label('output',1,'Out');
  PI with anti-windup and dynamic limits - Iq : Subsystem  mask(Discrete PI Controller with anti-windup and dynamic limiters){Kp=Q_Kp, Ki=Q_Ki, Init=0, Ts=Ts}
      mask prompts: Kp "Proportional gain (Kp):"; Ki "Integral gain (Ki):"; Init "State initial value:"; Ts "Sample time:"
      mask Display:
      | disp('PI-\nAST');
      | port_label('input',1,'Max');
      | port_label('input',2,'In');
      | port_label('input',3,'Min');
      | port_label('input',4,'Reset');
      | port_label('input',5,'x_reset');
      | port_label('output',1,'Out');
  PWM - average : Subsystem  mask{fboost=f_chopper, Ts=Ts}
      mask prompts: fboost "PWM frequency:"; Ts "Sample time (Ts):"
  Predictor1 : Subsystem  mask{Init_value=0, Ts=Ts}
      mask prompts: Init_value "Initial value:"; Ts "Sample time (Ts):"
  Predictor2 : Subsystem  mask{Init_value=0, Ts=Ts}
      mask prompts: Init_value "Initial value:"; Ts "Sample time (Ts):"
  Product{1..9} (9 alike) : Product
  Relay1 : Relay  OnSwitchValue=-(u_uvrt - frt_band)  OffSwitchValue=-(u_uvrt + frt_band)  OutDataTypeStr=Inherit: Inherit via back propagation
  Relay2 : Relay  OnSwitchValue=u_ovrt + frt_band  OffSwitchValue=u_ovrt - frt_band  OutDataTypeStr=Inherit: Inherit via back propagation
  Relay3 : Relay  OnSwitchValue=1.02*Vdc_ref  OffSwitchValue=1.015*Vdc_ref  OutDataTypeStr=Inherit: Inherit via back propagation
  Sample and Hold d : powerlib_meascontrol/Additional Components/Sample and Hold  ic=0  Ts=Ts
  Sample and Hold d1 : powerlib_meascontrol/Additional Components/Sample and Hold  ic=0  Ts=Ts
  Sample and Hold q : powerlib_meascontrol/Additional Components/Sample and Hold  ic=0  Ts=Ts
  Saturation Dynamic : simulink/Discontinuities/Saturation Dynamic  OutMin=[]  OutMax=[]  OutDataTypeStr=Inherit: Same as second input  OutDataType=fixdt(1, 16)  OutScaling=2^-10  DoSatur=off
  Saturation Dynamic1 : simulink/Discontinuities/Saturation Dynamic  OutMin=[]  OutMax=[]  OutDataTypeStr=Inherit: Same as second input  OutDataType=fixdt(1, 16)  OutScaling=2^-10  DoSatur=off
  Sqrt1 : Sqrt
  Sqrt2 : Sqrt
  Sum{1..2,4,13} (4 alike) : Sum  Inputs=|+-
  Sum11 : Sum  Inputs=|-+
  Sum12 : Sum  Inputs=+-|
  Sum14 : Sum  Inputs=-+|
  Sum5 : Sum  Inputs=|++
  Switch : Switch  Criteria=u2 > Threshold  Threshold=1.5  SaturateOnIntegerOverflow=off  InputSameDT=off
  Switch{1..3,5} (4 alike) : Switch  Criteria=u2 > Threshold  SaturateOnIntegerOverflow=off  InputSameDT=off
  Terminator3 : Terminator
  avoid neg i : Saturate  UpperLimit=i_max^2  LowerLimit=0
  avoid neg r : Saturate  UpperLimit=i_max^2  LowerLimit=0
  dq0 to abc : powerlib_meascontrol/Transformations/dq0 to abc  Alignment=90 degrees behind phase A axis
  k_uvrt1 : Gain  Gain=k_uvrt
  k_uvrt2 : Gain  Gain=k_ovrt
  max 1 : Saturate  UpperLimit=1  LowerLimit=0
  open breaker : Logic  Operator=NOR  AllPortsSameDT=off  OutDataTypeStr=boolean
  "pu -> A1" : Gain  Gain=i_rated
  "pu -> A2" : Gain  Gain=i_rated
  w_grid : Terminator
  i_ref : Outport
  ch_gate : Outport  Port=2
  protection : Outport  Port=3
  wires:
  Logical Operator5/1 -> Product6/1
  [UVRT] -> Logical Operator5/2
  [FRT_Mode1] -> Logical Operator5/1
  Q_ref/1 -> Discrete Transfer Fcn1/1, Discrete Transfer Fcn1/2
  Discrete Transfer Fcn1/1 -> [Q_ref_filt]
  Discrete Transfer Fcn4/1 -> [Q_meas_filt]
  Product7/1 -> Add1/2
  "pu -> A2"/1 -> Product7/1
  Logical Operator6/1 -> Product7/2
  [FRT_Mode1] -> Logical Operator6/2
  [OVRT] -> Logical Operator6/1
  Sum12/1 -> k_uvrt2/1
  k_uvrt2/1 -> "pu -> A2"/1
  Compare To Constant6/1 -> [FRT_Mode2]
  Constant15/1 -> Compare To Constant6/1
  Compare To Constant5/1 -> [FRT_Mode1]
  Constant14/1 -> Compare To Constant5/1
  [u_frt] -> Sum12/2
  Constant12/1 -> Sum12/1
  Add1/1 -> [di_imag_uvrt]
  Product6/1 -> Add1/1
  "pu -> A1"/1 -> Product6/2
  Sum11/1 -> k_uvrt1/1
  k_uvrt1/1 -> "pu -> A1"/1
  [u_frt] -> Sum11/1
  Constant9/1 -> Sum11/2
  Vdc_meas/1 -> [Vdc_meas], Discrete Transfer Fcn3/1
  dq0 to abc/1 -> i_ref/1
  Discrete Transfer Fcn3/1 -> [Vdc_filt]
  Mux8/1 -> dq0 to abc/1
  Product1/1 -> Mux8/1
  Constant21/1 -> Mux8/3
  [wt_ref] -> dq0 to abc/2
  Gain/1 -> Mux8/2
  Relay2/1 -> [OVRT], Logical Operator2/1
  Gain5/1 -> Relay1/1
  Relay1/1 -> Logical Operator2/2, [UVRT]
  u_frt/1 -> [u_frt], Relay2/1, Gain5/1
  Avoid FRT during initialization/1 -> [FRT_flag]
  0 ... 1/1 -> PWM - average/1(Duty-cycle)
  Constant5/1 -> Sum4/2
  Sum4/1 -> Gain2/1
  [Vdc_meas] -> Sum4/1
  Gain2/1 -> 0 ... 1/1
  PWM - average/1(gate) -> ch_gate/1
  avoid neg r/1 -> Sqrt1/1
  avoid neg i/1 -> Sqrt2/1
  [i_q] -> Math Function3/1
  [reac_prio] -> Switch2/2
  Sqrt2/1 -> Switch2/3
  Constant18/1 -> Switch2/1
  [reac_prio] -> Switch1/2
  Constant16/1 -> Switch1/3
  Sqrt1/1 -> Switch1/1
  [i_d] -> Math Function5/1
  Sum14/1 -> avoid neg i/1
  Constant11/1 -> Math Function4/1
  Sum13/1 -> avoid neg r/1
  Math Function3/1 -> Sum13/2
  Math Function2/1 -> Sum13/1
  Constant6/1 -> Math Function2/1
  Math Function4/1 -> Sum14/2
  Math Function5/1 -> Sum14/1
  Switch1/1 -> Switch3/3
  Switch3/1 -> Delay/1
  [id0_FRT2] -> Switch3/1
  [reset_id_FRT2] -> Switch3/2
  Switch2/1 -> Switch5/3
  [iq0_FRT2] -> Abs4/1
  [reset_iq_FRT2] -> Switch5/2
  Switch5/1 -> Delay1/1
  Delay/1 -> [i_d_lim]
  Delay1/1 -> [i_q_lim]
  Constant2/1 -> PI with anti-windup and dynamic limits - Id/3(LowerLimit)
  Sum2/1 -> Product4/2
  [Q_meas_filt] -> Sum1/2
  [Q_ref_filt] -> Sum1/1
  [i_q_lim] -> PI with anti-windup and dynamic limits - Iq/1(UpperLimit)
  Gain8/1 -> PI with anti-windup and dynamic limits - Iq/3(LowerLimit)
  Sum5/1 -> [i_q]
  [i_q_lim] -> Gain8/1
  [i_q_lim] -> Gain1/1
  [i_q_lim] -> Saturation Dynamic1/1
  Gain1/1 -> Saturation Dynamic1/3
  [i_d_lim] -> Saturation Dynamic/1
  Saturation Dynamic1/1 -> Delay3/1
  Saturation Dynamic/1 -> Delay2/1
  Constant4/1 -> Saturation Dynamic/3
  references/1 -> Demux1/1
  Demux1/2 -> [wt_ref]
  Demux1/1 -> [u_grid]
  Demux1/3 -> w_grid/1
  PQ_meas/1 -> Demux2/1
  [Vdc_filt] -> Sum2/1
  [i_d_lim] -> PI with anti-windup and dynamic limits - Id/1(UpperLimit)
  Constant1/1 -> Sum2/2
  Sum1/1 -> Product3/1
  Demux2/2 -> Discrete Transfer Fcn4/1
  Demux2/1 -> Terminator3/1
  Abs4/1 -> Switch5/1
  [FRT_flag] -> Compare To Constant/1
  Discrete-Time Integrator2/1 -> Compare To Constant3/1
  Data Type Conversion4/1 -> Discrete-Time Integrator2/2, Discrete-Time Integrator2/1
  Compare To Constant3/1 -> Counter AST/Trigger
  Counter AST/1(Count) -> max 1/1
  Compare To Constant/1 -> Data Type Conversion4/1
  max 1/1 -> open breaker/1
  u_f_protect/1 -> open breaker/2
  open breaker/1 -> [protection], protection/1
  [FRT_Mode2] -> Logical Operator4/1
  [FRT_flag] -> Logical Operator4/2
  [i_d] -> Delay d1/1
  [i_q] -> Delay q1/1
  Delay d1/1 -> Sample and Hold d1/1, Sample and Hold d/1
  Delay q1/1 -> Sample and Hold q/1
  Edge Detector1/1 -> Sample and Hold d/2, Sample and Hold q/2
  Constant13/1 -> Discrete-Time Integrator3/1
  Discrete-Time Integrator3/1 -> Compare To Constant7/1
  Compare To Constant7/1 -> Data Type Conversion1/1
  Product5/1 -> Predictor1/1(in)
  Product8/1 -> Predictor2/1(in)
  Sample and Hold q/1 -> Product8/1
  Predictor2/1(out) -> [iq0_FRT2]
  FRT_ramp_q/1(y) -> Compare To Constant9/1, Product8/2
  Compare To Constant9/1 -> [reset_iq_FRT2]
  FRT_ramp_p/1(y) -> Compare To Constant8/1, Product5/2
  [Vdc_filt] -> Relay3/1
  Compare To Constant8/1 -> Logical Operator11/1
  Logical Operator11/1 -> Logical Operator1/1
  Logical Operator4/1 -> Discrete-Time Integrator3/2, Logical Operator1/2, Edge Detector1/1
  Logical Operator1/1 -> [reset_id_FRT2]
  Data Type Conversion1/1 -> FRT_ramp_q/2(u), FRT_ramp_p/2(u)
  Relay3/1 -> Logical Operator11/2
  Constant19/1 -> FRT_ramp_p/1(UpperLimit)
  Constant20/1 -> FRT_ramp_p/3(LowerLimit)
  Constant22/1 -> FRT_ramp_q/1(UpperLimit)
  Constant23/1 -> FRT_ramp_q/3(LowerLimit)
  Switch/1 -> PI with anti-windup and dynamic limits - Id/5(x_reset)
  [FRT_Mode1] -> Logical Operator3/1
  [FRT_flag] -> Logical Operator3/2
  Logical Operator3/1 -> Edge Detector4/1, Edge Detector3/1, [reac_prio]
  Edge Detector3/1 -> Sample and Hold d1/2
  Sample and Hold d1/1 -> [id0_FRT1]
  Edge Detector4/1 -> Data Type Conversion2/1
  Data Type Conversion2/1 -> [reset_id_FRT1]
  [reset_id_FRT1] -> Logical Operator7/1
  [reset_id_FRT2] -> Logical Operator7/2
  Logical Operator7/1 -> PI with anti-windup and dynamic limits - Id/4(Reset)
  Constant7/1 -> Switch/2
  [id0_FRT1] -> Switch/3
  [id0_FRT2] -> Switch/1
  Predictor1/1(out) -> [id0_FRT2]
  [FRT_flag] -> Logical Operator8/1
  Logical Operator8/1 -> Product3/2
  [reset_iq_FRT2] -> PI with anti-windup and dynamic limits - Iq/4(Reset)
  [iq0_FRT2] -> PI with anti-windup and dynamic limits - Iq/5(x_reset)
  [di_imag_uvrt] -> Sum5/2
  PI with anti-windup and dynamic limits - Iq/1(Output) -> Sum5/1
  PI with anti-windup and dynamic limits - Id/1(Output) -> [i_d]
  Delay2/1 -> Product1/1
  Delay3/1 -> Product2/2
  [protection] -> Product2/1, Product1/2
  Product2/1 -> Gain/1
  Product4/1 -> PI with anti-windup and dynamic limits - Id/2(Input)
  [protection] -> Product4/1
  Product9/1 -> PI with anti-windup and dynamic limits - Iq/2(Input)
  Product3/1 -> Product9/2
  [protection] -> Product9/1
  [i_d] -> Saturation Dynamic/2
  [i_q] -> Saturation Dynamic1/2
  Sample and Hold d/1 -> Product5/1
  Logical Operator2/1 -> Avoid FRT during initialization/1
  Constant3/1 -> Avoid FRT during initialization/3
  Digital Clock2/1 -> Avoid FRT during initialization/2

== system WindTurbine_TypeIV_HM/Generic Type IV HM/Predictor1 ==
  in : Inport
  Delay : Delay  DelayLength=1  InitialCondition=Init_value  SampleTime=Ts
  Delay1 : Delay  DelayLength=1  InitialCondition=Init_value  SampleTime=Ts
  Gain : Gain  Gain=2
  Sum1 : Sum  Inputs=|+-
  out : Outport
  wires:
  in/1 -> Delay/1
  Delay1/1 -> Sum1/2
  Sum1/1 -> out/1
  Delay/1 -> Gain/1, Delay1/1
  Gain/1 -> Sum1/1

== system WindTurbine_TypeIV_HM/Generic Type IV HM/Predictor2 ==
  in : Inport
  Delay : Delay  DelayLength=1  InitialCondition=Init_value  SampleTime=Ts
  Delay1 : Delay  DelayLength=1  InitialCondition=Init_value  SampleTime=Ts
  Gain : Gain  Gain=2
  Sum1 : Sum  Inputs=|+-
  out : Outport
  wires:
  Gain/1 -> Sum1/1
  Delay/1 -> Delay1/1, Gain/1
  Sum1/1 -> out/1
  Delay1/1 -> Sum1/2
  in/1 -> Delay/1

== system WindTurbine_TypeIV_HM/Generic Type IV HM/Predictor4 ==
  in : Inport
  Delay : Delay  DelayLength=1  InitialCondition=Init_value  SampleTime=Ts
  Delay1 : Delay  DelayLength=1  InitialCondition=Init_value  SampleTime=Ts
  Gain : Gain  Gain=2
  Sum1 : Sum  Inputs=|+-
  out : Outport
  wires:
  Gain/1 -> Sum1/1
  Delay/1 -> Delay1/1, Gain/1
  Sum1/1 -> out/1
  Delay1/1 -> Sum1/2
  in/1 -> Delay/1
